simulink model "induction_motor"  (R2023b)
settings: Solver=VariableStepAuto  StartTime=0.0  StopTime=2  FixedStep=0.001  RelTol=1e-3
undefined symbols (not defined in the file or in its folder): J, K_r, L_m, L_s, R_s, T_r, Z_p
settings Model: Creator=anste  LastModifiedBy=anste

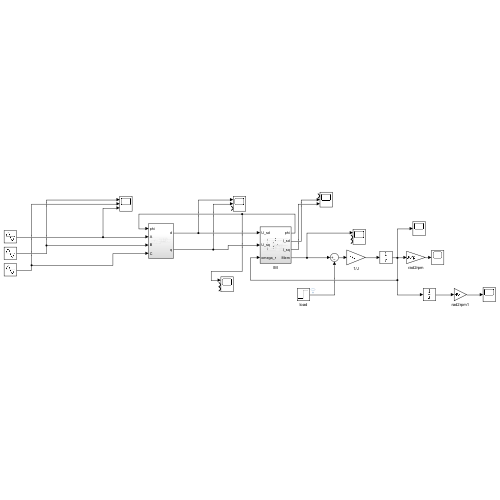
[thumbnail: Simulink's stored preview of the top-level diagram]
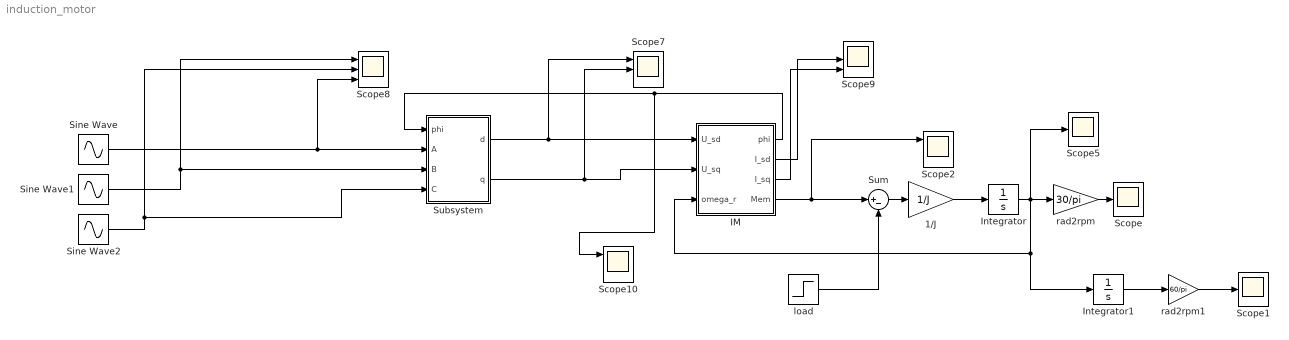
== system induction_motor ==
  1/J : Gain  Gain=1/J  SaturateOnIntegerOverflow=on  OutDataTypeStr=Inherit: Same as input  ParamDataTypeStr=Inherit: Same as input
  IM : Subsystem
  Integrator : Integrator
  Integrator1 : Integrator
  Scope : Scope
  Scope1 : Scope
  Scope{2,7..10} (5 alike) : Scope  NumInputPorts=3
  Scope5 : Scope
  Sine Wave : Sin  Amplitude=220  Frequency=50*2*pi  SampleTime=0
  Sine Wave1 : Sin  Amplitude=220  Frequency=50*2*pi  Phase=-2*pi/3  SampleTime=0
  Sine Wave2 : Sin  Amplitude=220  Frequency=50*2*pi  Phase=2*pi/3  SampleTime=0
  Subsystem : Subsystem
  Sum : Sum  Inputs=|+-
  load : Step  SampleTime=0
  rad2rpm : Gain  Gain=30/pi
  rad2rpm1 : Gain  Gain=60/pi
  wires:
  Integrator/1 -> Integrator1/1, IM/3(omega_r), Scope5/1, rad2rpm/1
  rad2rpm/1 -> Scope/1
  Sine Wave/1 -> Scope8/3, Subsystem/2(A)
  IM/1(phi) -> Scope10/1, Subsystem/1(phi)
  Subsystem/1(d) -> Scope7/1, IM/1(U_sd)
  Subsystem/2(q) -> Scope7/2, IM/2(U_sq)
  IM/4(Mem) -> Scope2/1, Sum/1
  1/J/1 -> Integrator/1
  Sum/1 -> 1/J/1
  Sine Wave2/1 -> Scope8/2, Subsystem/4(C)
  IM/2(I_sd) -> Scope9/2
  IM/3(I_sq) -> Scope9/3
  load/1 -> Sum/2
  Sine Wave1/1 -> Scope8/1, Subsystem/3(B)
  Integrator1/1 -> rad2rpm1/1
  rad2rpm1/1 -> Scope1/1

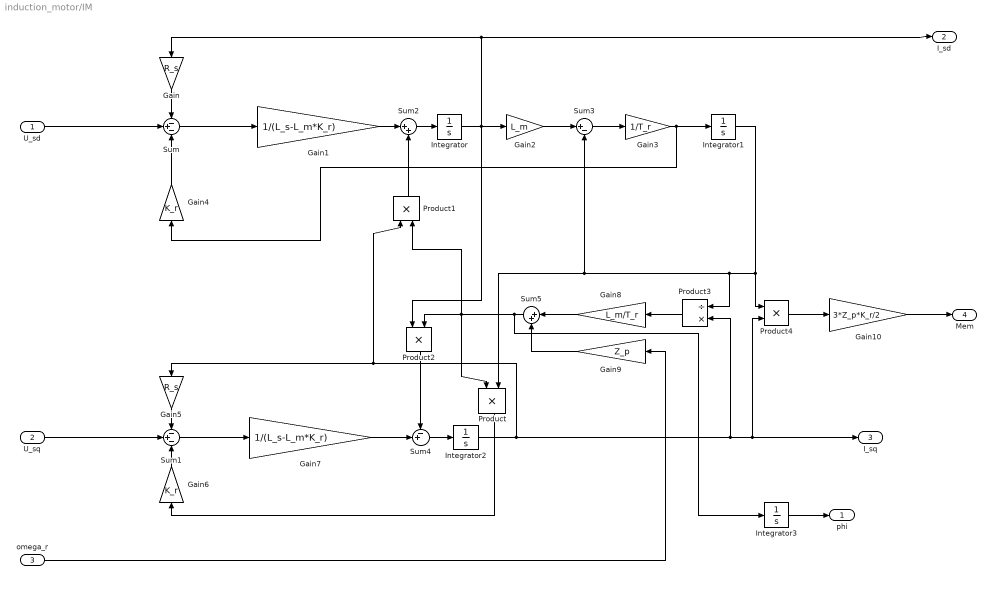
== system induction_motor/IM ==
  U_sd : Inport
  U_sq : Inport  Port=2
  omega_r : Inport  Port=3
  Gain : Gain  Gain=R_s
  Gain1 : Gain  Gain=1/(L_s-L_m*K_r)
  Gain10 : Gain  Gain=3*Z_p*K_r/2
  Gain2 : Gain  Gain=L_m
  Gain3 : Gain  Gain=1/T_r
  Gain4 : Gain  Gain=K_r
  Gain5 : Gain  Gain=R_s
  Gain6 : Gain  Gain=K_r
  Gain7 : Gain  Gain=1/(L_s-L_m*K_r)
  Gain8 : Gain  Gain=L_m/T_r
  Gain9 : Gain  Gain=Z_p
  Integrator : Integrator
  Integrator1 : Integrator  InitialCondition=1e-10
  Integrator2 : Integrator
  Integrator3 : Integrator
  Product : Product  Inputs=**
  Product1 : Product
  Product2 : Product
  Product3 : Product  Inputs=/*
  Product4 : Product
  Sum : Sum  Inputs=-+-
  Sum1 : Sum  Inputs=-+-
  Sum2 : Sum  Inputs=|++
  Sum3 : Sum  Inputs=|+-
  Sum4 : Sum  Inputs=-+|
  Sum5 : Sum  Inputs=|++
  phi : Outport
  I_sd : Outport  Port=2
  I_sq : Outport  Port=3
  Mem : Outport  Port=4
  wires:
  Gain9/1 -> Sum5/2
  Integrator2/1 -> Product3/2, Product4/2, I_sq/1, Product1/1, Gain5/1
  Sum2/1 -> Integrator/1
  Gain2/1 -> Sum3/1
  Sum4/1 -> Integrator2/1
  Sum5/1 -> Integrator3/1, Product/1, Product1/2, Product2/2
  Sum/1 -> Gain1/1
  Sum1/1 -> Gain7/1
  Sum3/1 -> Gain3/1
  Product/1 -> Gain6/1
  Gain/1 -> Sum/1
  Gain7/1 -> Sum4/2
  Gain10/1 -> Mem/1
  Gain3/1 -> Integrator1/1, Gain4/1
  Gain1/1 -> Sum2/1
  Integrator/1 -> Gain2/1, I_sd/1, Gain/1, Product2/1
  Gain4/1 -> Sum/3
  Gain5/1 -> Sum1/1
  Integrator1/1 -> Product4/1, Product3/1, Product/2, Sum3/2
  Product3/1 -> Gain8/1
  U_sq/1 -> Sum1/2
  Product2/1 -> Sum4/1
  Product4/1 -> Gain10/1
  Product1/1 -> Sum2/2
  Gain8/1 -> Sum5/1
  Gain6/1 -> Sum1/3
  U_sd/1 -> Sum/2
  omega_r/1 -> Gain9/1
  Integrator3/1 -> phi/1

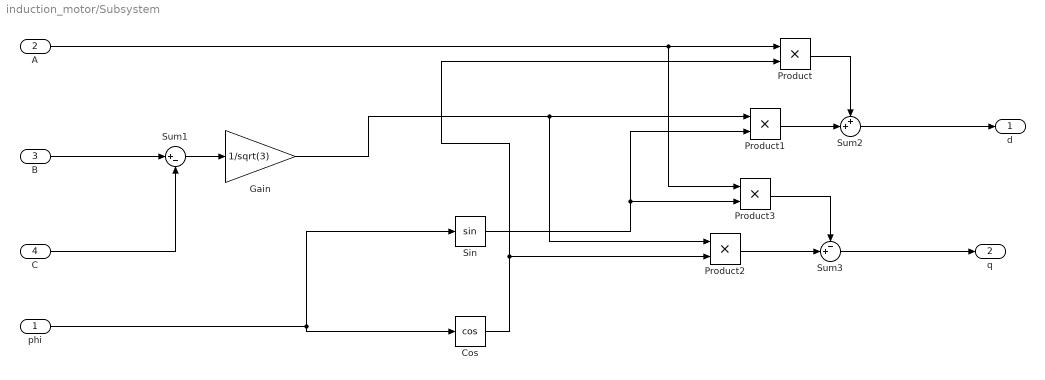
== system induction_motor/Subsystem ==
  phi : Inport
  A : Inport  Port=2
  B : Inport  Port=3
  C : Inport  Port=4
  Cos : Trigonometry  Operator=cos
  Gain : Gain  Gain=1/sqrt(3)
  Product{,1..3} (4 alike) : Product
  Sin : Trigonometry
  Sum1 : Sum  Inputs=|+-
  Sum2 : Sum  Inputs=++|
  Sum3 : Sum  Inputs=-+|
  d : Outport
  q : Outport  Port=2
  wires:
  phi/1 -> Sin/1, Cos/1
  Sum1/1 -> Gain/1
  Sum2/1 -> d/1
  C/1 -> Sum1/2
  B/1 -> Sum1/1
  Sum3/1 -> q/1
  A/1 -> Product3/1, Product/1
  Cos/1 -> Product2/2, Product/2
  Product/1 -> Sum2/1
  Product1/1 -> Sum2/2
  Gain/1 -> Product2/1, Product1/1
  Sin/1 -> Product3/2, Product1/2
  Product2/1 -> Sum3/2
  Product3/1 -> Sum3/1
